simulink model "MultiLoop_mode1"  (R2019a)
settings: Solver=ode1  StartTime=0.0  StopTime=24  FixedStep=Ts_base  MaxStep=Ts_base  MinStep=1e-6  RelTol=1e-6
PreLoadFcn:
  | addpath('..\sutils\RealTimeSlower')
InitFcn:
  | Mode_1_Init
StopFcn:
  | %TEplot
  | 
  | % date_string = datestr(now,'yyyymmdd-HHMM');
  | % save(['E:\TESTBED_MEASUREMENTS\TESIM\sim_out' date_string '.mat'],'sim_out')
undefined symbols (not defined in the file): r1_0, r4_0, Ts_base, Ts_save
libraries: TElib x17, TcAdsLib x6, utility x1
settings Model: Creator=rnc4  LastModifiedBy=rnc4
settings DataIOCC: LoadInitialState=on  SaveFinalState=on  SaveFormat=Structure  SignalLoggingSaveFormat=ModelDataLogs  SaveOutput=off  SaveTime=off  ReturnWorkspaceOutputs=off  SignalLoggingName=sigsOut
settings OptimizationCC: InitFltsAndDblsToZero=on  LifeSpan=inf
settings DebuggingCC: SaveWithParameterizedLinksMsg=none  UnderspecifiedInitializationDetection=Classic  MergeDetectMultiDrivingBlocksExec=none  SignalResolutionControl=TryResolveAllWithWarning  MultiTaskDSMMsg=warning  MultiTaskCondExecSysMsg=none  FcnCallInpInsideContextMsg=warning  SFUnexpectedBacktrackingDiag=warning  SFNoUnconditionalDefaultTransitionDiag=warning  ArithmeticOperatorsInVariantConditions=warning
settings HardwareCC: ProdBitPerPointer=32  ProdBitPerSizeT=32  ProdBitPerPtrDiffT=32  ProdLargestAtomicFloat=None  ProdIntDivRoundTo=Undefined  ProdEndianess=Unspecified  ProdWordSize=32  ProdHWDeviceType=32-bit Generic  TargetUnknown=on
settings ModelReferenceCC: PropagateSignalLabelsOutOfModel=off
settings SFSimCC: SimUseLocalCustomCode=off
settings RTWCC: RTWUseLocalCustomCode=off
settings CodeAppCC: StateflowObjectComments=on
settings GRTTargetCC: TargetFcnLib=ansi_tfl_tmw.mat  TargetLangStandard=C89/C90 (ANSI)  GeneratePreprocessorConditionals=Disable all  CombineOutputUpdateFcns=off  GRTInterface=on
settings ConfigComp: CovMetricSettings=dw  CovHtmlReporting=on  CovSaveCumulativeToWorkspaceVar=on  CovSaveSingleToWorkspaceVar=on  CovExternalEMLEnable=off

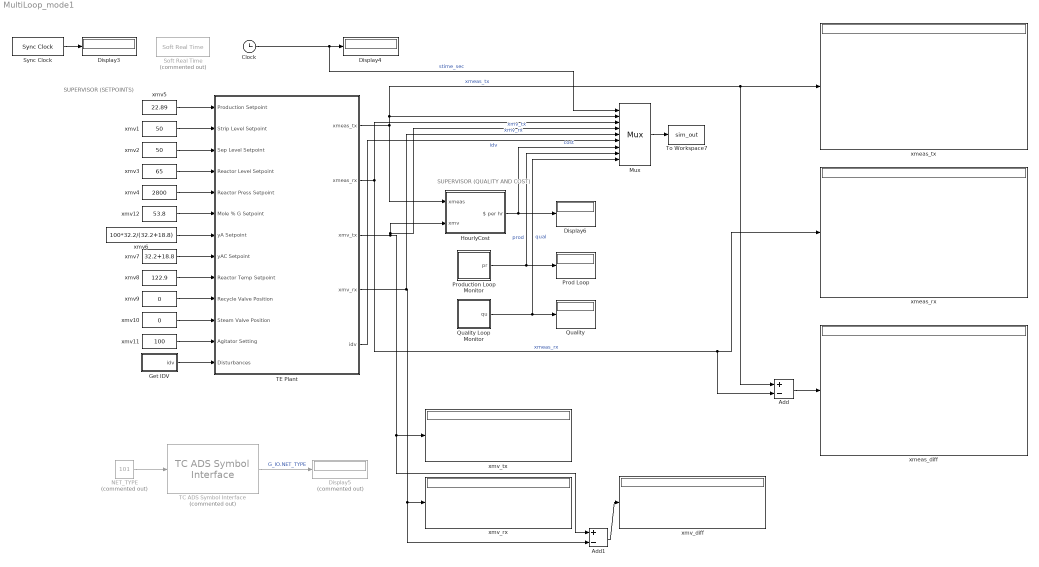
== system MultiLoop_mode1 ==
  note: SUPERVISOR (QUALITY AND COST)
  note: SUPERVISOR (SETPOINTS)
  Add : Sum  Inputs=+-
  Add1 : Sum  Inputs=+-
  Clock : Clock
  Display3 : Display
  Display4 : Display
  Display5 : Display  Commented=on
  Display6 : Display
  Get IDV : Subsystem
  HourlyCost : Subsystem
  Mux : Mux  Inputs=9
      settings: DisplayOption=signals
  NET_TYPE : Constant  Commented=on  Value=101  OutDataTypeStr=int32
  Prod Loop : Display
  Production Loop Monitor : Subsystem
  Quality : Display
  Quality Loop Monitor : Subsystem
  Soft Real Time : utility/Soft Real Time  Commented=on  x=3600
  Sync Clock : TcAdsLib/Utilities/Sync Clock  OutputPortSelect=System clock (t_clock)  InputPortSelect=None
      settings: SourceProductName=Beckhoff TwinCAT ADS Interface
  TC ADS Symbol Interface : TcAdsLib/Synchronous/TC ADS Symbol Interface  Commented=on  ConnectMode=1  TmiPathStorageMode=0  TargetAmsNetId=0.0.0.0.0.0  TargetModuleOid=0  SyncMode=0  TcTimeOutport=0  TimeStampOutport=0  SampleTime=0.0005  BufferLength=10  DelayTime=-1  Symbols_SimulinkToTwinCat=|  Symbols_TwinCatToSimulink=|  AdsErrorHandling=2  ChangeRowColOrder=on  CodeGenInputConnectType=DataArea (InputDst)  CodeGenOutputConnectType=DataArea (OutputSrc)
      Symbols_SimulinkToTwinCat=|
      | <?xml version="1.0" encoding="utf-8"?>
      | <SymbolAcquisitionInfoCollection xmlns:xsd="http://www.w3.org/2001/XMLSchema" xmlns:xsi="http://www.w3.org/2001/XMLSchema-instance">
      |   <SymbolInfos>
      |     <SymbolAcquisitionInfo>
      |       <Comment> specify network type
      |  100 					: ISA110.11a iMesh calibration
      |  101 					: ISA110.11a iMesh TESIM
      |  102 					: ISA110.11a iMesh test signals
      |  110					: ISA100.11a iMesh PN Sequence generation
      |  200 					: PhoenixContact calibration
      |  201					: PhoenixContact TESIM
      |  202					: PhoenixContact test signals
      |  210					: ISA100.11a PC OneLink PN Sequence generation</Comment>
      |       <Scope2Datatype>INT32</Scope2Datatype>
      |       <IndexGroup>16448</IndexGroup>
      |       <IndexOffset>384632</IndexOffset>
      |       <Name>G_IO.NET_TYPE</Name>
      |       <ShortName>NET_TYPE</ShortName>
      |       <Size>4</Size>
      |       <Type>DINT</Type>
      |       <TypeGUID>00000000-0000-0000-0000-000000000000</TypeGUID>
      |       <IsArray>false</IsArray>
      |       <ArrayLength>0</ArrayLength>
      |       <ConnectType>Symobl</ConnectType>
      |       <Datatype>ADST_INT32</Datatype>
      |       <NetId>5.53.143.24.1.1</NetId>
      |       <Port>851</Port>
      |       <SubSymbolCount>0</SubSymbolCount>
      |       <IsBitValue>false</IsBitValue>
      |       <IsPersistent>false</IsPersistent>
      |       <IsBitType>false</IsBitType>
      |       <IsPointer>false</IsPointer>
      |       <IsReadOnly>false</IsReadOnly>
      |       <IsReference>false</IsReference>
      |       <IsTcComInterfacePointer>false</IsTcComInterfacePointer>
      |       <IsTypeGuid>false</IsTypeGuid>
      |       <ContextMask>0</ContextMask>
      |       <Attributes>
      |         <ArrayOfSymbolAttribute />
      |       </Attributes>
      |       <DataTypeAttributes>
      |         <ArrayOfSymbolAttribute />
      |       </DataTypeAttributes>
      |     </SymbolAcquisitionInfo>
      |   </SymbolInfos>
      | </SymbolAcquisitionInfoCollection>
      Symbols_TwinCatToSimulink=|
      | <?xml version="1.0" encoding="utf-8"?>
      | <SymbolAcquisitionInfoCollection xmlns:xsd="http://www.w3.org/2001/XMLSchema" xmlns:xsi="http://www.w3.org/2001/XMLSchema-instance">
      |   <SymbolInfos>
      |     <SymbolAcquisitionInfo>
      |       <Comment> specify network type
      |  100 					: ISA110.11a iMesh calibration
      |  101 					: ISA110.11a iMesh TESIM
      |  102 					: ISA110.11a iMesh test signals
      |  110					: ISA100.11a iMesh PN Sequence generation
      |  200 					: PhoenixContact calibration
      |  201					: PhoenixContact TESIM
      |  202					: PhoenixContact test signals
      |  210					: ISA100.11a PC OneLink PN Sequence generation</Comment>
      |       <Scope2Datatype>INT32</Scope2Datatype>
      |       <IndexGroup>16448</IndexGroup>
      |       <IndexOffset>384632</IndexOffset>
      |       <Name>G_IO.NET_TYPE</Name>
      |       <ShortName>NET_TYPE</ShortName>
      |       <Size>4</Size>
      |       <Type>DINT</Type>
      |       <TypeGUID>00000000-0000-0000-0000-000000000000</TypeGUID>
      |       <IsArray>false</IsArray>
      |       <ArrayLength>0</ArrayLength>
      |       <ConnectType>Symobl</ConnectType>
      |       <Datatype>ADST_INT32</Datatype>
      |       <NetId>5.53.143.24.1.1</NetId>
      |       <Port>851</Port>
      |       <SubSymbolCount>0</SubSymbolCount>
      |       <IsBitValue>false</IsBitValue>
      |       <IsPersistent>false</IsPersistent>
      |       <IsBitType>false</IsBitType>
      |       <IsPointer>false</IsPointer>
      |       <IsReadOnly>false</IsReadOnly>
      |       <IsReference>false</IsReference>
      |       <IsTcComInterfacePointer>false</IsTcComInterfacePointer>
      |       <IsTypeGuid>false</IsTypeGuid>
      |       <ContextMask>0</ContextMask>
      |       <Attributes>
      |         <ArrayOfSymbolAttribute />
      |       </Attributes>
      |       <DataTypeAttributes>
      |         <ArrayOfSymbolAttribute />
      |       </DataTypeAttributes>
      |     </SymbolAcquisitionInfo>
      |   </SymbolInfos>
      | </SymbolAcquisitionInfoCollection>
      settings: SourceProductName=Beckhoff TwinCAT ADS Interface
  TE Plant : Subsystem
  To Workspace7 : ToWorkspace  VariableName=sim_out  SampleTime=Ts_save
  xmeas_diff : Display
  xmeas_rx : Display
  xmeas_tx : Display
  xmv1 : Constant  Value=50
  xmv10 : Constant  Value=0
  xmv11 : Constant  Value=100
  xmv12 : Constant  Value=53.8
  xmv2 : Constant  Value=50
  xmv3 : Constant  Value=65
  xmv4 : Constant  Value=2800
  xmv5 : Constant  Value=22.89
  xmv6 : Constant  Value=100*32.2/(32.2+18.8)
  xmv7 : Constant  Value=32.2+18.8
  xmv8 : Constant  Value=122.9
  xmv9 : Constant  Value=0
  xmv_diff : Display
  xmv_rx : Display
  xmv_tx : Display
  wires:
  xmv1/1 -> TE Plant/2(Strip Level Setpoint)
  xmv2/1 -> TE Plant/3(Sep Level Setpoint)
  xmv3/1 -> TE Plant/4(Reactor Level Setpoint)
  xmv4/1 -> TE Plant/5(Reactor Press Setpoint)
  xmv8/1 -> TE Plant/9(Reactor Temp Setpoint)
  xmv6/1 -> TE Plant/7(yA Setpoint)
  xmv7/1 -> TE Plant/8(yAC Setpoint)
  TE Plant/3(xmv_tx) -> Mux/4, HourlyCost/2(xmv), Add1/1, xmv_tx/1  "xmv_tx"
  TE Plant/5(idv) -> Mux/6  "idv"
  Clock/1 -> Mux/1, Display4/1  "stime_sec"
  HourlyCost/1($ per hr) -> Mux/7, Display6/1  "cost"
  xmv9/1 -> TE Plant/10(Recycle Valve Position)
  xmv10/1 -> TE Plant/11(Steam Valve Position)
  xmv11/1 -> TE Plant/12(Agitator Setting)
  xmv12/1 -> TE Plant/6(Mole % G Setpoint)
  xmv5/1 -> TE Plant/1(Production Setpoint)
  TE Plant/1(xmeas_tx) -> Add/1, xmeas_tx/1, Mux/2, HourlyCost/1(xmeas)  "xmeas_tx"
  Sync Clock/1 -> Display3/1
  NET_TYPE/1 -> TC ADS Symbol Interface/1
  TC ADS Symbol Interface/1 -> Display5/1  "G_IO.NET_TYPE"
  Production Loop Monitor/1(pr) -> Prod Loop/1, Mux/8  "prod"
  Quality Loop Monitor/1(qu) -> Mux/9, Quality/1  "qual"
  TE Plant/4(xmv_rx) -> Mux/5, Add1/2, xmv_rx/1  "xmv_rx"
  Mux/1 -> To Workspace7/1
  TE Plant/2(xmeas_rx) -> Mux/3, Add/2, xmeas_rx/1  "xmeas_rx"
  Get IDV/1(idv) -> TE Plant/13(Disturbances)
  Add/1 -> xmeas_diff/1
  Add1/1 -> xmv_diff/1

== system MultiLoop_mode1/Get IDV ==
  Data Type Conversion : DataTypeConversion  OutDataTypeStr=double
  Local_IDV : Constant  Value=zeros(20,1)
  Manual Switch : ManualSwitch
  TC ADS Symbol Interface1 : TcAdsLib/Synchronous/TC ADS Symbol Interface  ConnectMode=1  TmiPathStorageMode=0  TargetAmsNetId=0.0.0.0.0.0  TargetModuleOid=0  SyncMode=0  TcTimeOutport=0  TimeStampOutport=0  SampleTime=0.0005  BufferLength=10  DelayTime=-1  Symbols_SimulinkToTwinCat=|  Symbols_TwinCatToSimulink=|  AdsErrorHandling=2  ChangeRowColOrder=on  CodeGenInputConnectType=DataArea (InputDst)  CodeGenOutputConnectType=DataArea (OutputSrc)
      Symbols_SimulinkToTwinCat=|
      | <?xml version="1.0" encoding="utf-8"?>
      | <SymbolAcquisitionInfoCollection xmlns:xsd="http://www.w3.org/2001/XMLSchema" xmlns:xsi="http://www.w3.org/2001/XMLSchema-instance">
      |   <SymbolInfos />
      | </SymbolAcquisitionInfoCollection>
      Symbols_TwinCatToSimulink=|
      | <?xml version="1.0" encoding="utf-8"?>
      | <SymbolAcquisitionInfoCollection xmlns:xsd="http://www.w3.org/2001/XMLSchema" xmlns:xsi="http://www.w3.org/2001/XMLSchema-instance">
      |   <SymbolInfos>
      |     <SymbolAcquisitionInfo>
      |       <Comment> disturbances as set in tesim</Comment>
      |       <Scope2Datatype>INT32</Scope2Datatype>
      |       <IndexGroup>16448</IndexGroup>
      |       <IndexOffset>385688</IndexOffset>
      |       <Name>G_IO.IDV</Name>
      |       <ShortName>IDV</ShortName>
      |       <Size>80</Size>
      |       <Type>ARRAY [1..20] OF DINT</Type>
      |       <TypeGUID>00000000-0000-0000-0000-000000000000</TypeGUID>
      |       <IsArray>true</IsArray>
      |       <ArrayLength>20</ArrayLength>
      |       <ConnectType>Symobl</ConnectType>
      |       <Datatype>ADST_INT32</Datatype>
      |       <NetId>5.53.143.24.1.1</NetId>
      |       <Port>851</Port>
      |       <SubSymbolCount>0</SubSymbolCount>
      |       <IsBitValue>false</IsBitValue>
      |       <IsPersistent>false</IsPersistent>
      |       <IsBitType>false</IsBitType>
      |       <IsPointer>false</IsPointer>
      |       <IsReadOnly>false</IsReadOnly>
      |       <IsReference>false</IsReference>
      |       <IsTcComInterfacePointer>false</IsTcComInterfacePointer>
      |       <IsTypeGuid>false</IsTypeGuid>
      |       <ContextMask>0</ContextMask>
      |       <Attributes>
      |         <ArrayOfSymbolAttribute />
      |       </Attributes>
      |       <DataTypeAttributes>
      |         <ArrayOfSymbolAttribute />
      |       </DataTypeAttributes>
      |     </SymbolAcquisitionInfo>
      |   </SymbolInfos>
      | </SymbolAcquisitionInfoCollection>
      settings: SourceProductName=Beckhoff TwinCAT ADS Interface
  idv : Outport
  wires:
  TC ADS Symbol Interface1/1 -> Data Type Conversion/1  "G_IO.IDV"
  Data Type Conversion/1 -> Manual Switch/1
  Manual Switch/1 -> idv/1
  Local_IDV/1 -> Manual Switch/2

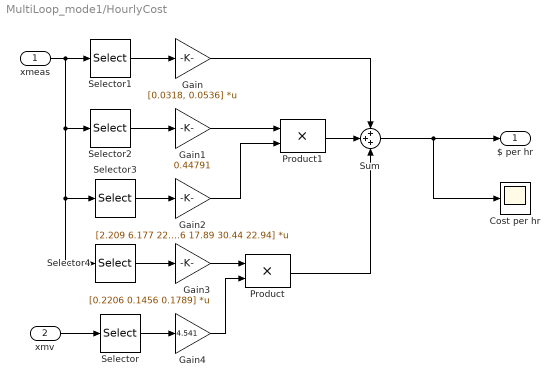
== system MultiLoop_mode1/HourlyCost ==
  xmeas : Inport  PortDimensions=41
  xmv : Inport  Port=2  PortDimensions=12
  Cost per hr : Scope
  Gain : Gain  Gain=[0.0318, 0.0536]  Multiplication=Matrix(K*u)  SaturateOnIntegerOverflow=on  OutDataTypeStr=Inherit: Same as input  ParamDataTypeStr=Inherit: Same as input
  Gain1 : Gain  Gain=0.44791  SaturateOnIntegerOverflow=on  OutDataTypeStr=Inherit: Same as input  ParamDataTypeStr=Inherit: Same as input
  Gain2 : Gain  Gain=[2.209 6.177 22.06 14.56 17.89 30.44 22.94]  Multiplication=Matrix(K*u)  SaturateOnIntegerOverflow=on  OutDataTypeStr=Inherit: Same as input  ParamDataTypeStr=Inherit: Same as input
  Gain3 : Gain  Gain=[0.2206 0.1456 0.1789]  Multiplication=Matrix(K*u)  SaturateOnIntegerOverflow=on  OutDataTypeStr=Inherit: Same as input  ParamDataTypeStr=Inherit: Same as input
  Gain4 : Gain  Gain=4.541  SaturateOnIntegerOverflow=on  OutDataTypeStr=Inherit: Same as input  ParamDataTypeStr=Inherit: Same as input
  Product : Product  SaturateOnIntegerOverflow=on  OutDataTypeStr=Inherit: Same as first input
  Product1 : Product  SaturateOnIntegerOverflow=on  OutDataTypeStr=Inherit: Same as first input
  Selector : Selector  InputPortWidth=12  IndexOptions=Index vector (dialog)  Indices=8  OutputSizes=1
  Selector1 : Selector  InputPortWidth=41  IndexOptions=Index vector (dialog)  Indices=[19 20]  OutputSizes=1
  Selector2 : Selector  InputPortWidth=41  IndexOptions=Index vector (dialog)  Indices=[10]  OutputSizes=1
  Selector3 : Selector  InputPortWidth=41  IndexOptions=Index vector (dialog)  Indices=[29, 31:36]  OutputSizes=1
  Selector4 : Selector  InputPortWidth=41  IndexOptions=Index vector (dialog)  Indices=[37:39]  OutputSizes=1
  Sum : Sum  Inputs=+++  SaturateOnIntegerOverflow=on
  $ per hr : Outport
  wires:
  xmv/1 -> Selector/1
  xmeas/1 -> Selector1/1, Selector2/1, Selector3/1, Selector4/1
  Selector1/1 -> Gain/1
  Selector2/1 -> Gain1/1
  Selector3/1 -> Gain2/1
  Selector4/1 -> Gain3/1
  Selector/1 -> Gain4/1
  Gain3/1 -> Product/1
  Gain4/1 -> Product/2
  Sum/1 -> Cost per hr/1, $ per hr/1
  Product/1 -> Sum/3
  Gain/1 -> Sum/1
  Product1/1 -> Sum/2
  Gain1/1 -> Product1/1
  Gain2/1 -> Product1/2

== system MultiLoop_mode1/Production Loop Monitor ==
  Mux2 : Mux  Inputs=2
  Production : Scope
  pr : Outport
  wires:
  Mux2/1 -> pr/1, Production/1
  [xmeas17] -> Mux2/2
  [Prodsp] -> Mux2/1

== system MultiLoop_mode1/Quality Loop Monitor ==
  Mux2 : Mux  Inputs=2
  Quality : Scope
  qu : Outport
  wires:
  [PctGsp] -> Mux2/1
  [xmeas40] -> Mux2/2
  Mux2/1 -> qu/1, Quality/1

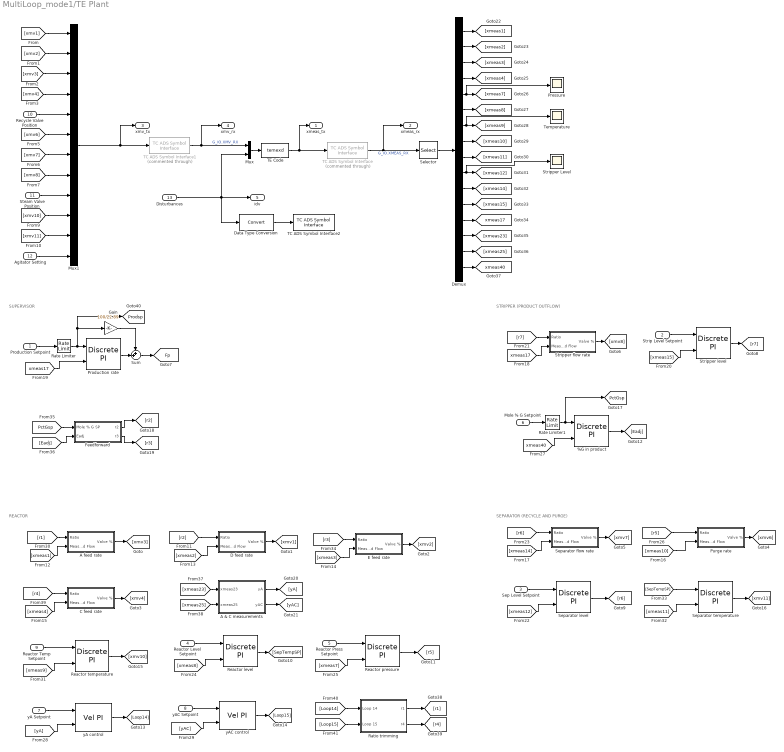
== system MultiLoop_mode1/TE Plant ==
  note: STRIPPER (PRODUCT OUTFLOW)
  note: SEPARATOR (RECYCLE AND PURGE)
  note: REACTOR
  note: SUPERVISOR
  Production Setpoint : Inport
  Strip Level Setpoint : Inport  Port=2
  Sep Level Setpoint : Inport  Port=3
  Reactor Level Setpoint : Inport  Port=4
  Reactor Press Setpoint : Inport  Port=5
  Mole % G Setpoint : Inport  Port=6
  yA Setpoint : Inport  Port=7
  yAC Setpoint : Inport  Port=8
  Reactor Temp Setpoint : Inport  Port=9
  Recycle Valve Position : Inport  Port=10
  Steam Valve Position : Inport  Port=11
  Agitator Setting : Inport  Port=12
  Disturbances : Inport  Port=13
  %G in product : TElib/Discrete PI  Kc=-0.4  Ti=100/60  Ts=Ts_base  x0=Eadj_0  Hi=inf  Lo=-inf
  A & C measurements : Subsystem
  A feed rate : Subsystem
  C feed rate : Subsystem
  D feed rate : Subsystem
  Data Type Conversion : DataTypeConversion
  Demux : Demux  Outputs=16
  E feed rate : Subsystem
  Feedforward : Subsystem
  Gain : Gain  Gain=100/22.89  SaturateOnIntegerOverflow=on  OutDataTypeStr=Inherit: Same as input  ParamDataTypeStr=Inherit: Same as input
  Mux : Mux  Inputs=2
  Mux1 : Mux  Inputs=12
  Pressure : Scope
  Production rate : TElib/Discrete PI  Kc=3.2  Ti=120/60  Ts=Ts_base  x0=0  Hi=30  Lo=-30
  Purge rate : Subsystem
  Rate Limiter : RateLimiter  RisingSlewLimit=0.3*22.95/24  FallingSlewLimit=-0.3*22.95/24
  Rate Limiter1 : RateLimiter  RisingSlewLimit=50/24  FallingSlewLimit=-50/24
  Ratio trimming : Subsystem
  Reactor level : TElib/Discrete PI  Kc=0.8  Ti=60/60  Ts=Ts_base  x0=SP17_0  Hi=120  Lo=0
  Reactor pressure : TElib/Discrete PI  Kc=-1e-4  Ti=20/60  Ts=Ts_base  x0=r5_0  Hi=100  Lo=0
  Reactor temperature : TElib/Discrete PI  Kc=-8  Ti=7.5/60  Ts=Ts_base  x0=xmv10_0  Hi=100  Lo=0
  Selector : Selector  InputPortWidth=41  IndexOptions=Index vector (dialog)  Indices=[1:4, 7:12, 14, 15, 17, 23, 25, 40]  OutputSizes=1
  Separator flow rate : Subsystem
  Separator level : TElib/Discrete PI  Kc=-1e-3  Ti=200/60  Ts=Ts_base  x0=r6_0  Hi=100  Lo=0
  Separator temperature : TElib/Discrete PI  Kc=-4  Ti=15/60  Ts=Ts_base  x0=xmv11_0  Hi=100  Lo=0
  Stripper Level : Scope
  Stripper flow rate : Subsystem
  Stripper level : TElib/Discrete PI  Kc=-2e-4  Ti=200/60  Ts=Ts_base  x0=r7_0  Hi=100  Lo=0
  Sum : Sum  Inputs=++|  SaturateOnIntegerOverflow=on
  TC ADS Symbol Interface : TcAdsLib/Synchronous/TC ADS Symbol Interface  Commented=through  ConnectMode=1  TmiPathStorageMode=0  TargetAmsNetId=0.0.0.0.0.0  TargetModuleOid=0  SyncMode=0  TcTimeOutport=0  TimeStampOutport=0  SampleTime=0.0005  BufferLength=10  DelayTime=-1  Symbols_SimulinkToTwinCat=|  Symbols_TwinCatToSimulink=|  AdsErrorHandling=2  ChangeRowColOrder=on  CodeGenInputConnectType=DataArea (InputDst)  CodeGenOutputConnectType=DataArea (OutputSrc)
      | <?xml version="1.0" encoding="utf-8"?>
      | <SymbolAcquisitionInfoCollection xmlns:xsd="http://www.w3.org/2001/XMLSchema" xmlns:xsi="http://www.w3.org/2001/XMLSchema-instance">
      |   <SymbolInfos>
      |     <SymbolAcquisitionInfo>
      |       <Comment> XMEAS reported by tesim</Comment>
      |       <Scope2Datatype>REAL64</Scope2Datatype>
      |       <IndexGroup>16448</IndexGroup>
      |       <IndexOffset>384696</IndexOffset>
      |       <Name>G_IO.XMEAS</Name>
      |       <ShortName>XMEAS</ShortName>
      |       <Size>328</Size>
      |       <Type>ARRAY [1..41] OF LREAL</Type>
      |       <TypeGUID>00000000-0000-0000-0000-000000000000</TypeGUID>
      |       <IsArray>true</IsArray>
      |       <ArrayLength>41</ArrayLength>
      |       <ConnectType>Symobl</ConnectType>
      |       <Datatype>ADST_REAL64</Datatype>
      |       <NetId>5.53.143.24.1.1</NetId>
      |       <Port>851</Port>
      |       <SubSymbolCount>0</SubSymbolCount>
      |       <IsBitValue>false</IsBitValue>
      |       <IsPersistent>false</IsPersistent>
      |       <IsBitType>false</IsBitType>
      |       <IsPointer>false</IsPointer>
      |       <IsReadOnly>false</IsReadOnly>
      |       <IsReference>false</IsReference>
      |       <IsTcComInterfacePointer>false</IsTcComInterfacePointer>
      |       <IsTypeGuid>false</IsTypeGuid>
      |       <ContextMask>0</ContextMask>
      |       <Attributes>
      |         <ArrayOfSymbolAttribute />
      |       </Attributes>
      |       <DataTypeAttributes>
      |         <ArrayOfSymbolAttribute />
      |       </DataTypeAttributes>
      |     </SymbolAcquisitionInfo>
      |   </SymbolInfos>
      | </SymbolAcquisitionInfoCollection>
      | <?xml version="1.0" encoding="utf-8"?>
      | <SymbolAcquisitionInfoCollection xmlns:xsd="http://www.w3.org/2001/XMLSchema" xmlns:xsi="http://www.w3.org/2001/XMLSchema-instance">
      |   <SymbolInfos>
      |     <SymbolAcquisitionInfo>
      |       <Comment />
      |       <Scope2Datatype>REAL64</Scope2Datatype>
      |       <IndexGroup>16448</IndexGroup>
      |       <IndexOffset>385024</IndexOffset>
      |       <Name>G_IO.XMEAS_RX</Name>
      |       <ShortName>XMEAS_RX</ShortName>
      |       <Size>328</Size>
      |       <Type>ARRAY [1..41] OF LREAL</Type>
      |       <TypeGUID>00000000-0000-0000-0000-000000000000</TypeGUID>
      |       <IsArray>true</IsArray>
      |       <ArrayLength>41</ArrayLength>
      |       <ConnectType>Symobl</ConnectType>
      |       <Datatype>ADST_REAL64</Datatype>
      |       <NetId>5.53.143.24.1.1</NetId>
      |       <Port>851</Port>
      |       <SubSymbolCount>0</SubSymbolCount>
      |       <IsBitValue>false</IsBitValue>
      |       <IsPersistent>false</IsPersistent>
      |       <IsBitType>false</IsBitType>
      |       <IsPointer>false</IsPointer>
      |       <IsReadOnly>false</IsReadOnly>
      |       <IsReference>false</IsReference>
      |       <IsTcComInterfacePointer>false</IsTcComInterfacePointer>
      |       <IsTypeGuid>false</IsTypeGuid>
      |       <ContextMask>0</ContextMask>
      |       <Attributes>
      |         <ArrayOfSymbolAttribute />
      |       </Attributes>
      |       <DataTypeAttributes>
      |         <ArrayOfSymbolAttribute />
      |       </DataTypeAttributes>
      |     </SymbolAcquisitionInfo>
      |   </SymbolInfos>
      | </SymbolAcquisitionInfoCollection>
      settings: SourceProductName=Beckhoff TwinCAT ADS Interface
  TC ADS Symbol Interface1 : TcAdsLib/Synchronous/TC ADS Symbol Interface  Commented=through  ConnectMode=1  TmiPathStorageMode=0  TargetAmsNetId=0.0.0.0.0.0  TargetModuleOid=0  SyncMode=0  TcTimeOutport=0  TimeStampOutport=0  SampleTime=0.0005  BufferLength=10  DelayTime=-1  Symbols_SimulinkToTwinCat=|  Symbols_TwinCatToSimulink=|  AdsErrorHandling=2  ChangeRowColOrder=on  CodeGenInputConnectType=DataArea (InputDst)  CodeGenOutputConnectType=DataArea (OutputSrc)
      | <?xml version="1.0" encoding="utf-8"?>
      | <SymbolAcquisitionInfoCollection xmlns:xsd="http://www.w3.org/2001/XMLSchema" xmlns:xsi="http://www.w3.org/2001/XMLSchema-instance">
      |   <SymbolInfos>
      |     <SymbolAcquisitionInfo>
      |       <Comment> XMV values reported by tesim</Comment>
      |       <Scope2Datatype>REAL64</Scope2Datatype>
      |       <IndexGroup>16448</IndexGroup>
      |       <IndexOffset>385400</IndexOffset>
      |       <Name>G_IO.XMV</Name>
      |       <ShortName>XMV</ShortName>
      |       <Size>96</Size>
      |       <Type>ARRAY [1..12] OF LREAL</Type>
      |       <TypeGUID>00000000-0000-0000-0000-000000000000</TypeGUID>
      |       <IsArray>true</IsArray>
      |       <ArrayLength>12</ArrayLength>
      |       <ConnectType>Symobl</ConnectType>
      |       <Datatype>ADST_REAL64</Datatype>
      |       <NetId>5.53.143.24.1.1</NetId>
      |       <Port>851</Port>
      |       <SubSymbolCount>0</SubSymbolCount>
      |       <IsBitValue>false</IsBitValue>
      |       <IsPersistent>false</IsPersistent>
      |       <IsBitType>false</IsBitType>
      |       <IsPointer>false</IsPointer>
      |       <IsReadOnly>false</IsReadOnly>
      |       <IsReference>false</IsReference>
      |       <IsTcComInterfacePointer>false</IsTcComInterfacePointer>
      |       <IsTypeGuid>false</IsTypeGuid>
      |       <ContextMask>0</ContextMask>
      |       <Attributes>
      |         <ArrayOfSymbolAttribute />
      |       </Attributes>
      |       <DataTypeAttributes>
      |         <ArrayOfSymbolAttribute />
      |       </DataTypeAttributes>
      |     </SymbolAcquisitionInfo>
      |   </SymbolInfos>
      | </SymbolAcquisitionInfoCollection>
      | <?xml version="1.0" encoding="utf-8"?>
      | <SymbolAcquisitionInfoCollection xmlns:xsd="http://www.w3.org/2001/XMLSchema" xmlns:xsi="http://www.w3.org/2001/XMLSchema-instance">
      |   <SymbolInfos>
      |     <SymbolAcquisitionInfo>
      |       <Comment />
      |       <Scope2Datatype>REAL64</Scope2Datatype>
      |       <IndexGroup>16448</IndexGroup>
      |       <IndexOffset>385496</IndexOffset>
      |       <Name>G_IO.XMV_RX</Name>
      |       <ShortName>XMV_RX</ShortName>
      |       <Size>96</Size>
      |       <Type>ARRAY [1..12] OF LREAL</Type>
      |       <TypeGUID>00000000-0000-0000-0000-000000000000</TypeGUID>
      |       <IsArray>true</IsArray>
      |       <ArrayLength>12</ArrayLength>
      |       <ConnectType>Symobl</ConnectType>
      |       <Datatype>ADST_REAL64</Datatype>
      |       <NetId>5.53.143.24.1.1</NetId>
      |       <Port>851</Port>
      |       <SubSymbolCount>0</SubSymbolCount>
      |       <IsBitValue>false</IsBitValue>
      |       <IsPersistent>false</IsPersistent>
      |       <IsBitType>false</IsBitType>
      |       <IsPointer>false</IsPointer>
      |       <IsReadOnly>false</IsReadOnly>
      |       <IsReference>false</IsReference>
      |       <IsTcComInterfacePointer>false</IsTcComInterfacePointer>
      |       <IsTypeGuid>false</IsTypeGuid>
      |       <ContextMask>0</ContextMask>
      |       <Attributes>
      |         <ArrayOfSymbolAttribute />
      |       </Attributes>
      |       <DataTypeAttributes>
      |         <ArrayOfSymbolAttribute />
      |       </DataTypeAttributes>
      |     </SymbolAcquisitionInfo>
      |   </SymbolInfos>
      | </SymbolAcquisitionInfoCollection>
      settings: SourceProductName=Beckhoff TwinCAT ADS Interface
  TC ADS Symbol Interface2 : TcAdsLib/Synchronous/TC ADS Symbol Interface  ConnectMode=1  TmiPathStorageMode=0  TargetAmsNetId=0.0.0.0.0.0  TargetModuleOid=0  SyncMode=0  TcTimeOutport=0  TimeStampOutport=0  SampleTime=0.0005  BufferLength=10  DelayTime=-1  Symbols_SimulinkToTwinCat=|  Symbols_TwinCatToSimulink=|  AdsErrorHandling=2  ChangeRowColOrder=on  CodeGenInputConnectType=DataArea (InputDst)  CodeGenOutputConnectType=DataArea (OutputSrc)
      | <?xml version="1.0" encoding="utf-8"?>
      | <SymbolAcquisitionInfoCollection xmlns:xsd="http://www.w3.org/2001/XMLSchema" xmlns:xsi="http://www.w3.org/2001/XMLSchema-instance">
      |   <SymbolInfos>
      |     <SymbolAcquisitionInfo>
      |       <Comment> disturbances as set in tesim</Comment>
      |       <Scope2Datatype>INT32</Scope2Datatype>
      |       <IndexGroup>16448</IndexGroup>
      |       <IndexOffset>385688</IndexOffset>
      |       <Name>G_IO.IDV</Name>
      |       <ShortName>IDV</ShortName>
      |       <Size>80</Size>
      |       <Type>ARRAY [1..20] OF DINT</Type>
      |       <TypeGUID>00000000-0000-0000-0000-000000000000</TypeGUID>
      |       <IsArray>true</IsArray>
      |       <ArrayLength>20</ArrayLength>
      |       <ConnectType>Symobl</ConnectType>
      |       <Datatype>ADST_INT32</Datatype>
      |       <NetId>5.53.143.24.1.1</NetId>
      |       <Port>851</Port>
      |       <SubSymbolCount>0</SubSymbolCount>
      |       <IsBitValue>false</IsBitValue>
      |       <IsPersistent>false</IsPersistent>
      |       <IsBitType>false</IsBitType>
      |       <IsPointer>false</IsPointer>
      |       <IsReadOnly>false</IsReadOnly>
      |       <IsReference>false</IsReference>
      |       <IsTcComInterfacePointer>false</IsTcComInterfacePointer>
      |       <IsTypeGuid>false</IsTypeGuid>
      |       <ContextMask>0</ContextMask>
      |       <Attributes>
      |         <ArrayOfSymbolAttribute />
      |       </Attributes>
      |       <DataTypeAttributes>
      |         <ArrayOfSymbolAttribute />
      |       </DataTypeAttributes>
      |     </SymbolAcquisitionInfo>
      |   </SymbolInfos>
      | </SymbolAcquisitionInfoCollection>
      | <?xml version="1.0" encoding="utf-8"?>
      | <SymbolAcquisitionInfoCollection xmlns:xsd="http://www.w3.org/2001/XMLSchema" xmlns:xsi="http://www.w3.org/2001/XMLSchema-instance">
      |   <SymbolInfos />
      | </SymbolAcquisitionInfoCollection>
      settings: SourceProductName=Beckhoff TwinCAT ADS Interface
  TE Code : S-Function  FunctionName=temexd  Parameters=[]  SFunctionDeploymentMode=off  EnableBusSupport=off
  Temperature : Scope
  yA control : TElib/Discrete PI/Vel PI  Kc=2e-4  Ti=1  Ts=0.1
  yAC control : TElib/Discrete PI/Vel PI  Kc=3e-4  Ti=2  Ts=0.1
  xmeas_tx : Outport
  xmeas_rx : Outport  Port=2
  xmv_tx : Outport  Port=3
  xmv_rx : Outport  Port=4
  idv : Outport  Port=5
  tag scope: Fp=global, PctGsp=global, Prodsp=global, xmeas17=global, xmeas40=global
  wires:
  Mux/1 -> TE Code/1
  Disturbances/1 -> Data Type Conversion/1, idv/1, Mux/2
  [xmv1] -> Mux1/1
  [xmv2] -> Mux1/2
  [xmv3] -> Mux1/3
  [xmv4] -> Mux1/4
  Recycle Valve Position/1 -> Mux1/5
  [xmv6] -> Mux1/6
  [xmv7] -> Mux1/7
  [xmv8] -> Mux1/8
  Steam Valve Position/1 -> Mux1/9
  [xmv10] -> Mux1/10
  [xmv11] -> Mux1/11
  Agitator Setting/1 -> Mux1/12
  A feed rate/1(Valve %) -> [xmv3]
  [xmeas1] -> A feed rate/2(Measured Flow)
  D feed rate/1(Valve %) -> [xmv1]
  [xmeas2] -> D feed rate/2(Measured Flow)
  E feed rate/1(Valve %) -> [xmv2]
  [xmeas3] -> E feed rate/2(Measured Flow)
  C feed rate/1(Valve %) -> [xmv4]
  [xmeas4] -> C feed rate/2(Measured Flow)
  Purge rate/1(Valve %) -> [xmv6]
  [xmeas10] -> Purge rate/2(Measured Flow)
  Separator flow rate/1(Valve %) -> [xmv7]
  [xmeas14] -> Separator flow rate/2(Measured Flow)
  Stripper flow rate/1(Valve %) -> [xmv8]
  [xmeas17] -> Stripper flow rate/2(Measured Flow)
  [xmeas17] -> Production rate/2
  [xmeas15] -> Stripper level/2
  Strip Level Setpoint/1 -> Stripper level/1
  Stripper level/1 -> [r7]
  [r7] -> Stripper flow rate/1(Ratio)
  [xmeas12] -> Separator level/2
  Sep Level Setpoint/1 -> Separator level/1
  Separator level/1 -> [r6]
  [r6] -> Separator flow rate/1(Ratio)
  [xmeas8] -> Reactor level/2
  Reactor Level Setpoint/1 -> Reactor level/1
  Reactor level/1 -> [SepTempSP]
  [xmeas7] -> Reactor pressure/2
  Reactor Press Setpoint/1 -> Reactor pressure/1
  Reactor pressure/1 -> [r5]
  [r5] -> Purge rate/1(Ratio)
  [xmeas40] -> %G in product/2
  %G in product/1 -> [Eadj]
  [yA] -> yA control/2
  yA Setpoint/1 -> yA control/1
  yA control/1 -> [Loop14]
  [yAC] -> yAC control/2
  yAC Setpoint/1 -> yAC control/1
  yAC control/1 -> [Loop15]
  [r1] -> A feed rate/1(Ratio)
  [xmeas9] -> Reactor temperature/2
  Reactor Temp Setpoint/1 -> Reactor temperature/1
  Reactor temperature/1 -> [xmv10]
  [xmeas11] -> Separator temperature/2
  [SepTempSP] -> Separator temperature/1
  Separator temperature/1 -> [xmv11]
  [r2] -> D feed rate/1(Ratio)
  [r3] -> E feed rate/1(Ratio)
  [PctGsp] -> Feedforward/1(Mole % G SP)
  [Eadj] -> Feedforward/2(Eadj)
  Feedforward/1(r2) -> [r2]
  Feedforward/2(r3) -> [r3]
  [xmeas23] -> A & C measurements/1(xmeas23)
  [xmeas25] -> A & C measurements/2(xmeas25)
  A & C measurements/1(yA) -> [yA]
  A & C measurements/2(yAC) -> [yAC]
  Mux1/1 -> TC ADS Symbol Interface1/1, xmv_tx/1
  Selector/1 -> Demux/1
  Demux/1 -> [xmeas1]
  Demux/2 -> [xmeas2]
  Demux/3 -> [xmeas3]
  Demux/4 -> [xmeas4]
  Demux/5 -> [xmeas7], Pressure/1
  Demux/6 -> [xmeas8]
  Demux/7 -> [xmeas9], Temperature/1
  Demux/8 -> [xmeas10]
  Demux/9 -> [xmeas11]
  Demux/10 -> [xmeas12], Stripper Level/1
  Demux/11 -> [xmeas14]
  Demux/12 -> [xmeas15]
  Demux/13 -> [xmeas17]
  Demux/14 -> [xmeas23]
  Demux/15 -> [xmeas25]
  Demux/16 -> [xmeas40]
  [r4] -> C feed rate/1(Ratio)
  [Loop14] -> Ratio trimming/1(Loop 14)
  [Loop15] -> Ratio trimming/2(Loop 15)
  Ratio trimming/1(r1) -> [r1]
  Ratio trimming/2(r4) -> [r4]
  Production Setpoint/1 -> Rate Limiter/1
  Rate Limiter/1 -> Production rate/1, [Prodsp], Gain/1
  Mole % G Setpoint/1 -> Rate Limiter1/1
  Rate Limiter1/1 -> [PctGsp], %G in product/1
  Production rate/1 -> Sum/2
  Sum/1 -> [Fp]
  Gain/1 -> Sum/1
  TE Code/1 -> TC ADS Symbol Interface/1, xmeas_tx/1
  TC ADS Symbol Interface/1 -> xmeas_rx/1, Selector/1  "G_IO.XMEAS_RX"
  TC ADS Symbol Interface1/1 -> xmv_rx/1, Mux/1  "G_IO.XMV_RX"
  Data Type Conversion/1 -> TC ADS Symbol Interface2/1

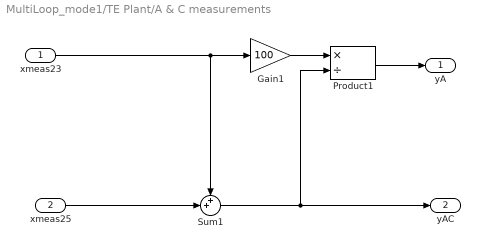
== system MultiLoop_mode1/TE Plant/A & C measurements ==
  xmeas23 : Inport
  xmeas25 : Inport  Port=2
  Gain1 : Gain  Gain=100  SaturateOnIntegerOverflow=on  OutDataTypeStr=Inherit: Same as input  ParamDataTypeStr=Inherit: Same as input
  Product1 : Product  Inputs=*/  SaturateOnIntegerOverflow=on  OutDataTypeStr=Inherit: Same as first input
  Sum1 : Sum  Inputs=++|  SaturateOnIntegerOverflow=on
  yA : Outport
  yAC : Outport  Port=2
  wires:
  Sum1/1 -> yAC/1, Product1/2
  xmeas23/1 -> Sum1/1, Gain1/1
  xmeas25/1 -> Sum1/2
  Gain1/1 -> Product1/1
  Product1/1 -> yA/1

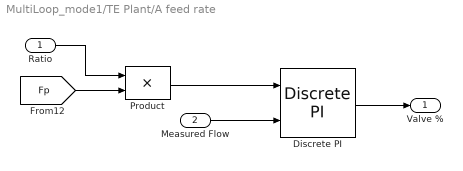
== system MultiLoop_mode1/TE Plant/A feed rate ==
  Ratio : Inport
  Measured Flow : Inport  Port=2
  Discrete PI : TElib/Discrete PI  Kc=0.01  Ti=0.001/60  Ts=Ts_base  x0=xmv3_0  Hi=100  Lo=0
  Product : Product  SaturateOnIntegerOverflow=on  OutDataTypeStr=Inherit: Same as first input
  Valve % : Outport
  wires:
  Discrete PI/1 -> Valve %/1
  Ratio/1 -> Product/1
  [Fp] -> Product/2
  Measured Flow/1 -> Discrete PI/2
  Product/1 -> Discrete PI/1

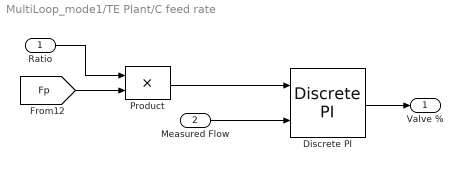
== system MultiLoop_mode1/TE Plant/C feed rate ==
  Ratio : Inport
  Measured Flow : Inport  Port=2
  Discrete PI : TElib/Discrete PI  Kc=0.003  Ti=0.001/60  Ts=Ts_base  x0=xmv4_0  Hi=100  Lo=0
  Product : Product  SaturateOnIntegerOverflow=on  OutDataTypeStr=Inherit: Same as first input
  Valve % : Outport
  wires:
  Product/1 -> Discrete PI/1
  Measured Flow/1 -> Discrete PI/2
  [Fp] -> Product/2
  Ratio/1 -> Product/1
  Discrete PI/1 -> Valve %/1

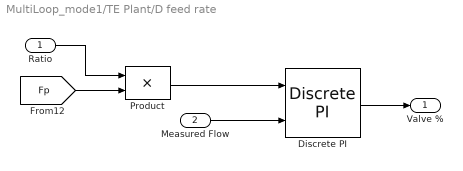
== system MultiLoop_mode1/TE Plant/D feed rate ==
  Ratio : Inport
  Measured Flow : Inport  Port=2
  Discrete PI : TElib/Discrete PI  Kc=1.6e-6  Ti=0.001/60  Ts=Ts_base  x0=xmv1_0  Hi=100  Lo=0
  Product : Product  SaturateOnIntegerOverflow=on  OutDataTypeStr=Inherit: Same as first input
  Valve % : Outport
  wires:
  Product/1 -> Discrete PI/1
  Measured Flow/1 -> Discrete PI/2
  [Fp] -> Product/2
  Ratio/1 -> Product/1
  Discrete PI/1 -> Valve %/1

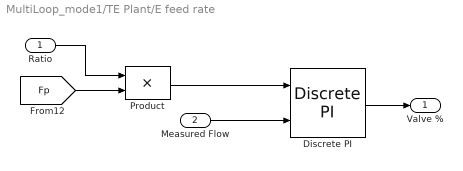
== system MultiLoop_mode1/TE Plant/E feed rate ==
  Ratio : Inport
  Measured Flow : Inport  Port=2
  Discrete PI : TElib/Discrete PI  Kc=1.8e-6  Ti=0.001/60  Ts=Ts_base  x0=xmv2_0  Hi=100  Lo=0
  Product : Product  SaturateOnIntegerOverflow=on  OutDataTypeStr=Inherit: Same as first input
  Valve % : Outport
  wires:
  Product/1 -> Discrete PI/1
  Measured Flow/1 -> Discrete PI/2
  [Fp] -> Product/2
  Ratio/1 -> Product/1
  Discrete PI/1 -> Valve %/1

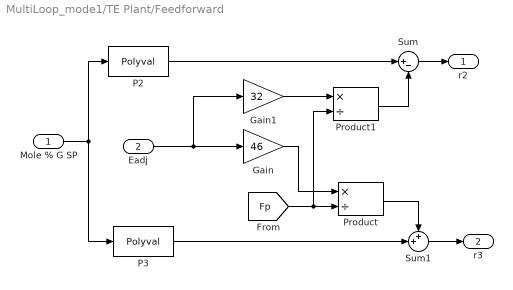
== system MultiLoop_mode1/TE Plant/Feedforward ==
  Mole % G SP : Inport
  Eadj : Inport  Port=2
  Gain : Gain  Gain=46  SaturateOnIntegerOverflow=on  OutDataTypeStr=Inherit: Same as input  ParamDataTypeStr=Inherit: Same as input
  Gain1 : Gain  Gain=32  SaturateOnIntegerOverflow=on  OutDataTypeStr=Inherit: Same as input  ParamDataTypeStr=Inherit: Same as input
  P2 : Polyval  Coefs="[1.5192e-003  5.9446e-001  2.7690e-001]"
  P3 : Polyval  Coefs="[-1.1377e-003 -8.0893e-001  9.1060e+001]"
  Product : Product  Inputs=*/  SaturateOnIntegerOverflow=on  OutDataTypeStr=Inherit: Same as first input
  Product1 : Product  Inputs=*/  SaturateOnIntegerOverflow=on  OutDataTypeStr=Inherit: Same as first input
  Sum : Sum  Inputs=|+-  SaturateOnIntegerOverflow=on
  Sum1 : Sum  Inputs=++|  SaturateOnIntegerOverflow=on
  r2 : Outport
  r3 : Outport  Port=2
  wires:
  Mole % G SP/1 -> P2/1, P3/1
  Sum/1 -> r2/1
  P2/1 -> Sum/1
  Sum1/1 -> r3/1
  P3/1 -> Sum1/2
  Product/1 -> Sum1/1
  [Fp] -> Product/2, Product1/2
  Gain/1 -> Product/1
  Eadj/1 -> Gain/1, Gain1/1
  Product1/1 -> Sum/2
  Gain1/1 -> Product1/1

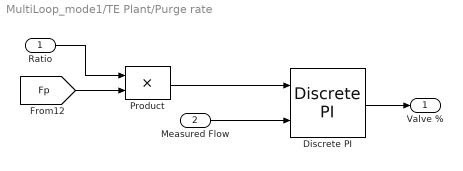
== system MultiLoop_mode1/TE Plant/Purge rate ==
  Ratio : Inport
  Measured Flow : Inport  Port=2
  Discrete PI : TElib/Discrete PI  Kc=0.01  Ti=0.001/60  Ts=Ts_base  x0=xmv6_0  Hi=100  Lo=0
  Product : Product  SaturateOnIntegerOverflow=on  OutDataTypeStr=Inherit: Same as first input
  Valve % : Outport
  wires:
  Discrete PI/1 -> Valve %/1
  Ratio/1 -> Product/1
  [Fp] -> Product/2
  Measured Flow/1 -> Discrete PI/2
  Product/1 -> Discrete PI/1

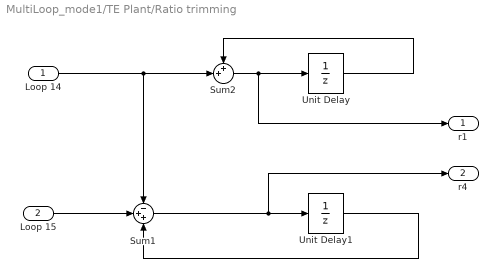
== system MultiLoop_mode1/TE Plant/Ratio trimming ==
  Loop 14 : Inport
  Loop 15 : Inport  Port=2
  Sum1 : Sum  Inputs=-++  SaturateOnIntegerOverflow=on
  Sum2 : Sum  Inputs=++|  SaturateOnIntegerOverflow=on
  Unit Delay : UnitDelay  InitialCondition=r1_0  SampleTime=0.1  HasFrameUpgradeWarning=on
  Unit Delay1 : UnitDelay  InitialCondition=r4_0  SampleTime=0.1  HasFrameUpgradeWarning=on
  r1 : Outport
  r4 : Outport  Port=2
  wires:
  Loop 15/1 -> Sum1/2
  Unit Delay/1 -> Sum2/1
  Unit Delay1/1 -> Sum1/3
  Sum2/1 -> Unit Delay/1, r1/1
  Loop 14/1 -> Sum2/2, Sum1/1
  Sum1/1 -> Unit Delay1/1, r4/1

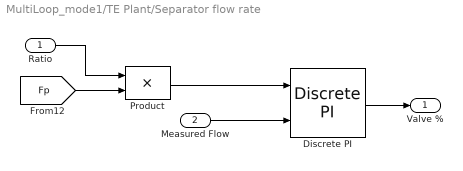
== system MultiLoop_mode1/TE Plant/Separator flow rate ==
  Ratio : Inport
  Measured Flow : Inport  Port=2
  Discrete PI : TElib/Discrete PI  Kc=4e-4  Ti=0.001/60  Ts=Ts_base  x0=xmv7_0  Hi=100  Lo=0
  Product : Product  SaturateOnIntegerOverflow=on  OutDataTypeStr=Inherit: Same as first input
  Valve % : Outport
  wires:
  Product/1 -> Discrete PI/1
  Measured Flow/1 -> Discrete PI/2
  [Fp] -> Product/2
  Ratio/1 -> Product/1
  Discrete PI/1 -> Valve %/1

== system MultiLoop_mode1/TE Plant/Stripper flow rate ==
  Ratio : Inport
  Measured Flow : Inport  Port=2
  Discrete PI : TElib/Discrete PI  Kc=4e-4  Ti=0.001/60  Ts=Ts_base  x0=xmv8_0  Hi=100  Lo=0
  Product : Product  SaturateOnIntegerOverflow=on  OutDataTypeStr=Inherit: Same as first input
  Valve % : Outport
  wires:
  Discrete PI/1 -> Valve %/1
  Ratio/1 -> Product/1
  [Fp] -> Product/2
  Measured Flow/1 -> Discrete PI/2
  Product/1 -> Discrete PI/1
